simulink model "CCModel_73"  (R2024a)
settings: Solver=ode3  StartTime=0.0  StopTime=100  FixedStep=0.001  RelTol=1e-3  EnableMultiTasking=on
undefined symbols (not defined in the file or in its folder): DiscIntNeverNeededParam, Hecate_desVel1, Hecate_desVel2, Hecate_desVel3, Hecate_horShift, Hecate_period, Hecate_slope, Hecate_Transition1, Hecate_Transition2, Hecate_verShift, i, PME_qb, qb_map, RPM_qb, V
libraries: simulink x46
(part 3 of 11)

== system CCModel_73/Powertrain/EMR ==
  note: If Torque is positive: Motor does its best
      | If torque is negative: Case 01: SOC > 99: No Regen (Tmot = 0)
      | Case 02: SOC < 99: Regen
      | If Vehicle is stopped: No Regen Brakes
  0 : Constant
  "1 " : Constant  Value=0
  EMS Active : Constant  Value=EMRActive
  GEN Ratio : Constant
  Memory1 : Memory  InheritSampleTime=on
  Negative Motor Torque Table : Lookup_n-D  NumberOfTableDimensions=1  BreakpointsForDimension1=|  Table=|  InternalRulePriority=Speed  RndMeth=Simplest
      BreakpointsForDimension1=|
      | [1
      | 300
      | 700
      | 1000
      | 1300
      | 1600
      | 1900
      | 2200
      | 2500
      | 2800
      | 3100
      | 3400
      | 3700
      | 4000
      | 4300
      | 4600
      | 4900
      | 5200
      | 5500
      | 5800
      | 6100
      | 6400
      | 6700
      | 7000
      | 7400
      | 7800
      | 8200
      | 8600
      | 8810]
      Table=|
      | [-360
      | -360
      | -360
      | -360
      | -360
      | -357.728404316261
      | -357.682405078656
      | -356.960983702214
      | -356.300227986961
      | -355.518140949330
      | -355.472141711725
      | -351.285699987009
      | -343.284814075766
      | -334.455149023278
      | -326.397812480700
      | -307.963362459085
      | -289.161940741908
      | -276.934802218937
      | -265.691686602383
      | -254.400604378871
      | -242.676261199004
      | -229.462130210989
      | -218.075437684875
      | -207.776256300937
      | -192.222891861329
      | -178.005775209291
      | -168.578005975641
      | -157.192637101830
      | -152.195121951219]
  Positive Motor Torque Table : Lookup_n-D  NumberOfTableDimensions=1  BreakpointsForDimension1=|  Table=|  InternalRulePriority=Speed  RndMeth=Simplest
      BreakpointsForDimension1=|
      | [1
      | 300
      | 700
      | 1000
      | 1300
      | 1600
      | 1900
      | 2200
      | 2500
      | 2800
      | 3100
      | 3400
      | 3700
      | 4000
      | 4300
      | 4600
      | 4900
      | 5200
      | 5500
      | 5800
      | 6100
      | 6400
      | 6700
      | 7000
      | 7400
      | 7800
      | 8200
      | 8600
      | 8810]
      Table=|
      | [360
      | 360
      | 360
      | 360
      | 360
      | 357.728404316261
      | 357.682405078656
      | 356.960983702214
      | 356.300227986961
      | 355.518140949330
      | 355.472141711725
      | 351.285699987009
      | 343.284814075766
      | 334.455149023278
      | 326.397812480700
      | 307.963362459085
      | 289.161940741908
      | 276.934802218937
      | 265.691686602383
      | 254.400604378871
      | 242.676261199004
      | 229.462130210989
      | 218.075437684875
      | 207.776256300937
      | 192.222891861329
      | 178.005775209291
      | 168.578005975641
      | 157.192637101830
      | 152.195121951219]
  Product : Product
  Saturation Dynamic1 : simulink/Discontinuities/Saturation Dynamic  OutMin=[-360]  OutMax=[360]  OutDataTypeStr=Inherit: Same as second input  OutDataType=fixdt(1, 16)  OutScaling=2^-10  DoSatur=off
  Switch : Switch  Criteria=u2 > Threshold  SaturateOnIntegerOverflow=off  InputSameDT=off
  Switch3 : Switch  SaturateOnIntegerOverflow=off  InputSameDT=off
  efficiency : Subsystem
  prod : Product
  prod1 : Product
  prod2 : Product
  rad_sec_to_rpm : Gain  Gain=60/2/pi
  tag scope: EMRRatio=global, EMRTorque=global, EMR_ElectricPower_W=global, InternalEMRActivity=global
  wires:
  [EMRTorqueCmd] -> Saturation Dynamic1/2
  Switch3/1 -> prod/1
  Positive Motor Torque Table/1 -> Saturation Dynamic1/1
  Product/1 -> [EMRTorque]
  "1 "/1 -> Switch/1
  [EMROutputOmega] -> rad_sec_to_rpm/1
  0/1 -> Switch/3
  prod/1 -> efficiency/2("Torque [Nm] "), Product/1
  EMS Active/1 -> prod1/2, prod/2, Switch/2
  GEN Ratio/1 -> [EMRRatio], Product/2
  Saturation Dynamic1/1 -> prod2/1, Switch3/2, Switch3/1
  Memory1/1 -> Negative Motor Torque Table/1, Positive Motor Torque Table/1
  Negative Motor Torque Table/1 -> Saturation Dynamic1/3
  rad_sec_to_rpm/1 -> efficiency/1(Motor speed [rpm]), Memory1/1
  prod1/1 -> [EMR_ElectricPower_W]
  efficiency/1(Electrical power [W]) -> prod1/1
  Switch/1 -> [InternalEMRActivity]
  [RegenFactor] -> prod2/2
  prod2/1 -> Switch3/3

== system CCModel_73/Powertrain/EMS ==
  note: If Torque is positive: Motor does its best
      | If torque is negative: Case 01: SOC > 99: No Regen (Tmot = 0)
      | Case 02: SOC < 99: Regen
      | If Vehicle is stopped: No Regen Brakes
  0 : Constant
  "1 " : Constant  Value=0
  Constant1 : Constant  Value=0
  EMS Active : Constant  Value=EMSActive
  GEN Ratio : Constant
  Memory1 : Memory  InheritSampleTime=on
  Negative Motor Torque Table : Lookup_n-D  NumberOfTableDimensions=1  BreakpointsForDimension1=|  Table=|  InternalRulePriority=Speed  RndMeth=Simplest
      BreakpointsForDimension1=|
      | [1
      | 300
      | 700
      | 1000
      | 1300
      | 1600
      | 1900
      | 2200
      | 2500
      | 2800
      | 3100
      | 3400
      | 3700
      | 4000
      | 4300
      | 4600
      | 4900
      | 5200
      | 5500
      | 5800
      | 6100
      | 6400
      | 6700
      | 7000
      | 7400
      | 7800
      | 8200
      | 8600
      | 8810]
      Table=|
      | [-360
      | -360
      | -360
      | -360
      | -360
      | -357.728404316261
      | -357.682405078656
      | -356.960983702214
      | -356.300227986961
      | -355.518140949330
      | -355.472141711725
      | -351.285699987009
      | -343.284814075766
      | -334.455149023278
      | -326.397812480700
      | -307.963362459085
      | -289.161940741908
      | -276.934802218937
      | -265.691686602383
      | -254.400604378871
      | -242.676261199004
      | -229.462130210989
      | -218.075437684875
      | -207.776256300937
      | -192.222891861329
      | -178.005775209291
      | -168.578005975641
      | -157.192637101830
      | -152.195121951219]
  Positive Motor Torque Table : Lookup_n-D  NumberOfTableDimensions=1  BreakpointsForDimension1=|  Table=|  InternalRulePriority=Speed  RndMeth=Simplest
      BreakpointsForDimension1=|
      | [1
      | 300
      | 700
      | 1000
      | 1300
      | 1600
      | 1900
      | 2200
      | 2500
      | 2800
      | 3100
      | 3400
      | 3700
      | 4000
      | 4300
      | 4600
      | 4900
      | 5200
      | 5500
      | 5800
      | 6100
      | 6400
      | 6700
      | 7000
      | 7400
      | 7800
      | 8200
      | 8600
      | 8810]
      Table=|
      | [360
      | 360
      | 360
      | 360
      | 360
      | 357.728404316261
      | 357.682405078656
      | 356.960983702214
      | 356.300227986961
      | 355.518140949330
      | 355.472141711725
      | 351.285699987009
      | 343.284814075766
      | 334.455149023278
      | 326.397812480700
      | 307.963362459085
      | 289.161940741908
      | 276.934802218937
      | 265.691686602383
      | 254.400604378871
      | 242.676261199004
      | 229.462130210989
      | 218.075437684875
      | 207.776256300937
      | 192.222891861329
      | 178.005775209291
      | 168.578005975641
      | 157.192637101830
      | 152.195121951219]
  Product : Product
  Saturation Dynamic1 : simulink/Discontinuities/Saturation Dynamic  OutMin=[-360]  OutMax=[360]  OutDataTypeStr=Inherit: Same as second input  OutDataType=fixdt(1, 16)  OutScaling=2^-10  DoSatur=off
  Switch : Switch  Criteria=u2 > Threshold  SaturateOnIntegerOverflow=off  InputSameDT=off
  Switch3 : Switch  SaturateOnIntegerOverflow=off  InputSameDT=off
  compare SOC to SOC _max : Switch  Criteria=u2 > Threshold  Threshold=99  SaturateOnIntegerOverflow=off  InputSameDT=off
  efficiency : Subsystem
  prod : Product
  prod1 : Product
  rad_sec_to_rpm : Gain  Gain=60/2/pi
  tag scope: EMSRatio=global, EMSTorque=global, EMS_ElectricPower_W=global, InternalEMSActivity=global
  wires:
  Switch/1 -> [InternalEMSActivity]
  "1 "/1 -> Switch/1
  0/1 -> Switch/3
  prod/1 -> efficiency/2("Torque [Nm] "), Product/1
  rad_sec_to_rpm/1 -> efficiency/1(Motor speed [rpm]), Memory1/1
  [EMSOutputOmega] -> rad_sec_to_rpm/1
  prod1/1 -> [EMS_ElectricPower_W]
  Negative Motor Torque Table/1 -> Saturation Dynamic1/3
  Product/1 -> [EMSTorque]
  GEN Ratio/1 -> [EMSRatio], Product/2
  Memory1/1 -> Negative Motor Torque Table/1, Positive Motor Torque Table/1
  Switch3/1 -> prod/1
  efficiency/1(Electrical power [W]) -> prod1/1
  Saturation Dynamic1/1 -> Switch3/2, Switch3/1, compare SOC to SOC _max/3
  [SOC] -> compare SOC to SOC _max/2
  compare SOC to SOC _max/1 -> Switch3/3
  Constant1/1 -> compare SOC to SOC _max/1
  Positive Motor Torque Table/1 -> Saturation Dynamic1/1
  EMS Active/1 -> prod1/2, prod/2, Switch/2
  [EMSTorqueCmd] -> Saturation Dynamic1/2

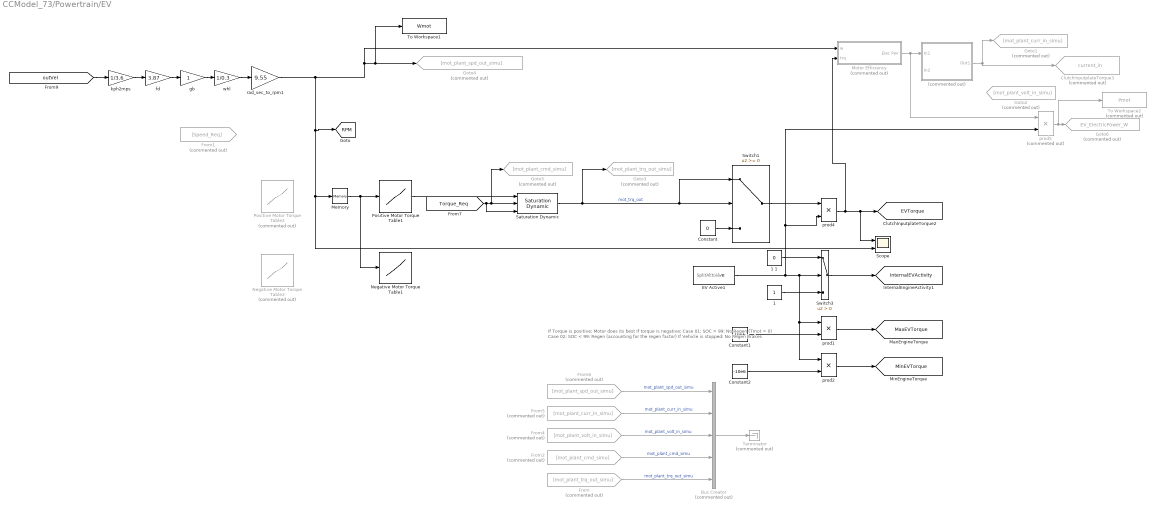
== system CCModel_73/Powertrain/EV ==
  note: If Torque is positive: Motor does its best
      | If torque is negative: Case 01: SOC > 99: No Regen (Tmot = 0)
      | Case 02: SOC < 99: Regen (accounting for the regen factor)
      | If Vehicle is stopped: No Regen Brakes
  note: SplitActive
  " " : Subsystem  Commented=on
      mask Display: fprintf('Divider')
  1 : Constant
  1 1 : Constant  Value=0
  Bus Creator : BusCreator  Commented=on  Inputs='mot_plant_spd_out_simu','mot_plant_curr_in_simu','mot_plant_volt_in_simu','mot_plant_cmd_simu','mot_plant_trq_out_simu'
  ClutchInputplateTorque3 : Goto  Commented=on  GotoTag=current_in  TagVisibility=global
  Constant : Constant  Value=0
  Constant1 : Constant  Value=10e6
  Constant2 : Constant  Value=-10e6
  EV Active1 : Constant  Value=EVActive
  From : From  Commented=on  GotoTag=mot_plant_trq_out_simu
  From1 : From  Commented=on  GotoTag=Speed_Req  TagVisibility=global
  From2 : From  Commented=on  GotoTag=mot_plant_cmd_simu
  From4 : From  Commented=on  GotoTag=mot_plant_volt_in_simu
  From5 : From  Commented=on  GotoTag=mot_plant_curr_in_simu
  From6 : From  Commented=on  GotoTag=mot_plant_spd_out_simu
  Goto1 : Goto  Commented=on  GotoTag=mot_plant_curr_in_simu
  Goto2 : Goto  Commented=on  GotoTag=mot_plant_volt_in_simu
  Goto3 : Goto  Commented=on  GotoTag=mot_plant_trq_out_simu
  Goto4 : Goto  Commented=on  GotoTag=mot_plant_spd_out_simu
  Goto5 : Goto  Commented=on  GotoTag=mot_plant_cmd_simu
  Goto6 : Goto  Commented=on  GotoTag=EV_ElectricPower_W  TagVisibility=global
  Memory : Memory
  Motor Efficiency : Subsystem  Commented=on
  Negative Motor Torque Table1 : Lookup_n-D  NumberOfTableDimensions=1  BreakpointsForDimension1="[5.65\t554.29\t1108.59\t1662.89\t2024.88\t2211.53\t2369.9\t2522.62\t2680.99\t2873.3\t3088.23\t3252.26\t3433.25\t3625.56\t3812.21\t4095.02\t4389.14\t4536.19\t4626.69\t4700.22\t4756.78\t4819\t4869.9\t4920.81\t4977.37\t4999.99]"  Table="[-444\t-444\t-444\t-444\t-428\t-416.41\t-396.47\t-372.36\t-344.93\t-310.84\t-285.92\t-268.48\t-248.55\t-233.62\t-218.68\t-200.45\t-193.05\t-186.44\t-173.14\t-154.84\t-129.037\t-101.56\t-73.26\t-46.62\t-17.48\t0]"  InternalRulePriority=Speed  RndMeth=Simplest
  Negative Motor Torque Table2 : Lookup_n-D  Commented=on  NumberOfTableDimensions=1  BreakpointsForDimension1=[0 5000]  Table=[-500 -500]  InternalRulePriority=Speed  RndMeth=Simplest
  Positive Motor Torque Table1 : Lookup_n-D  NumberOfTableDimensions=1  BreakpointsForDimension1=[1;10;575;750;925;1100;1275;1450;1625;1800;1975;2150;2325;2500;2675;2850;3025;3200;3375;3550;3725;3900;4075;4250;4425;4600;4775;4950;5125;5300;5475;5650;5825;6000]  Table=[412.5;412.5;412.5;412.5;412.5;412.5;412.5;412.5;412.5;412.5;412.5;412.5;412.5;412.5;412.5;412.5;412.5;412.5;412.5;412.5;400;380;355.5626875;346.30825;338.1746875;331.162;325.2701875;320.49925;316.8491875;314.32;308;275;50;0.195]  InternalRulePriority=Speed  RndMeth=Simplest
  Positive Motor Torque Table2 : Lookup_n-D  Commented=on  NumberOfTableDimensions=1  BreakpointsForDimension1=[0 500 1000 1500 2000 2500 3000 3500 4000 4500 5000]  Table=[436 426 416 408 405 330 258 207 172 140 0]  InternalRulePriority=Speed  RndMeth=Simplest
  Saturation Dynamic : simulink/Discontinuities/Saturation Dynamic  OutMin=[-444]  OutMax=[444]  OutDataTypeStr=Inherit: Same as second input  OutDataType=fixdt(1, 16)  OutScaling=2^-10  DoSatur=off
  Scope : Scope  NumInputPorts=2
  Switch1 : Switch  SaturateOnIntegerOverflow=off  InputSameDT=off
  Switch3 : Switch  Criteria=u2 > Threshold  SaturateOnIntegerOverflow=off  InputSameDT=off
  Terminator : Terminator  Commented=on
  To Workspace1 : ToWorkspace  VariableName=Wmot  SampleTime=-1
      settings: Save2DSignal=2-D array (concatenate along first dimension)
  To Workspace2 : ToWorkspace  Commented=on  VariableName=Pmot  SampleTime=-1
      settings: Save2DSignal=2-D array (concatenate along first dimension)
  fd : Gain  Gain=3.87
  gb : Gain
  kph2mps : Gain  Gain=1/3.6
  prod1 : Product
  prod2 : Product
  prod4 : Product
  prod5 : Product  Commented=on
  rad_sec_to_rpm1 : Gain  Gain=9.55
  whl : Gain  Gain=1/0.3
  tag scope: EVTorque=global, InternalEVActivity=global, MaxEVTorque=global, MinEVTorque=global, RPM=global
  wires:
  rad_sec_to_rpm1/1 -> [RPM], Scope/2, Memory/1, Motor Efficiency/1(w), To Workspace1/1, Goto4/1
  Saturation Dynamic/1 -> Switch1/2, Switch1/1, Goto3/1  "mot_trq_out"
  From5/1 -> Bus Creator/2  "mot_plant_curr_in_simu"
  [Torque_Req] -> Saturation Dynamic/3, Goto5/1, Saturation Dynamic/2
  From/1 -> Bus Creator/5  "mot_plant_trq_out_simu"
  Bus Creator/1 -> Terminator/1
  From6/1 -> Bus Creator/1  "mot_plant_spd_out_simu"
  Memory/1 -> Negative Motor Torque Table1/1, Positive Motor Torque Table1/1
  Positive Motor Torque Table1/1 -> Saturation Dynamic/1
  From2/1 -> Bus Creator/4  "mot_plant_cmd_simu"
  From4/1 -> Bus Creator/3  "mot_plant_volt_in_simu"
  [outVel] -> kph2mps/1
  1 1/1 -> Switch3/1
  Switch3/1 -> [InternalEVActivity]
  1/1 -> Switch3/3
  Switch1/1 -> prod4/1
  prod5/1 -> To Workspace2/1, Goto6/1
  Motor Efficiency/1(Elec Pwr) -> prod5/1, " "/1(In1)
  " "/1(Out1) -> ClutchInputplateTorque3/1, Goto1/1
  Constant2/1 -> prod2/2
  EV Active1/1 -> prod5/2, prod4/2, prod1/1, prod2/1, Switch3/2
  Constant1/1 -> prod1/2
  fd/1 -> gb/1
  gb/1 -> whl/1
  kph2mps/1 -> fd/1
  whl/1 -> rad_sec_to_rpm1/1
  prod4/1 -> Motor Efficiency/2(trq), Scope/1, [EVTorque]
  prod1/1 -> [MaxEVTorque]
  prod2/1 -> [MinEVTorque]
  Constant/1 -> Switch1/3

== system CCModel_73/Powertrain/Engine ==
  1 2 : Constant  Value=0
  2 : Constant
  Constant1 : Constant  Value=10e6
  Constant2 : Constant  Value=-10e6
  Eengine Active : Constant  Value=EngineActive
  EngineOmega : Goto  Commented=on  GotoTag=EngineOmega  TagVisibility=global
  Fuel Consumption : Subsystem  Commented=on
      mask Display: image(imread('engine_icon.jpg'))
  ICE_WOT : Lookup_n-D  NumberOfTableDimensions=1  BreakpointsForDimension1=[0 1500 2000 2500 3000 3500 4000 4500 5000 5500 6000 6500 7000 7200]  Table=[0 460 475 490 500 510 530 540 530 510 480 455 420 400]  InternalRulePriority=Speed  RndMeth=Simplest
  IdleSpeed(rpm) : Constant  Value=IdleSpeed
  Idle_Speed : Saturate  UpperLimit=inf  LowerLimit=800
  Idle_if_N : Switch  Criteria=u2 > Threshold  SaturateOnIntegerOverflow=off  InputSameDT=off
  Memory18 : Memory  InheritSampleTime=on
  Memory2 : Memory  InheritSampleTime=on
  Min : MinMax  Inputs=2
  Product6 : Product
  Saturation : Saturate  UpperLimit=inf  LowerLimit=0
  Switch1 : Switch  Criteria=u2 > Threshold  SaturateOnIntegerOverflow=off  InputSameDT=off
  prod{1..4} (4 alike) : Product
  rad_sec_to_rpm2 : Gain  Gain=60/2/pi
  rpm_to_radsec : Gain  Gain=1/(60/2/pi)
  tag scope: ClutchInputplateTorque=global, InternalEngineActivity=global, MaxEngineTorque=global, MinEngineTorque=global
  wires:
  Constant1/1 -> prod1/2
  Constant2/1 -> prod2/2
  [EngineTorqueCmd] -> Min/1
  prod3/1 -> [ClutchInputplateTorque]
  Eengine Active/1 -> prod4/2, prod3/2, prod2/1, prod1/1, Switch1/2
  ICE_WOT/1 -> Min/2
  1 2/1 -> Switch1/1
  2/1 -> Switch1/3
  rad_sec_to_rpm2/1 -> Memory2/1
  Switch1/1 -> [InternalEngineActivity]
  Saturation/1 -> prod3/1
  Min/1 -> Saturation/1
  Idle_Speed/1 -> ICE_WOT/1
  Memory2/1 -> Idle_Speed/1
  Memory18/1 -> prod4/1, rad_sec_to_rpm2/1
  prod1/1 -> [MaxEngineTorque]
  prod2/1 -> [MinEngineTorque]
  [DiffCenterInputOmega] -> Product6/2
  [GearRatio] -> Idle_if_N/2, Product6/1
  Product6/1 -> Idle_if_N/1
  prod4/1 -> EngineOmega/1
  Idle_if_N/1 -> Memory18/1
  IdleSpeed(rpm)/1 -> rpm_to_radsec/1
  rpm_to_radsec/1 -> Idle_if_N/3

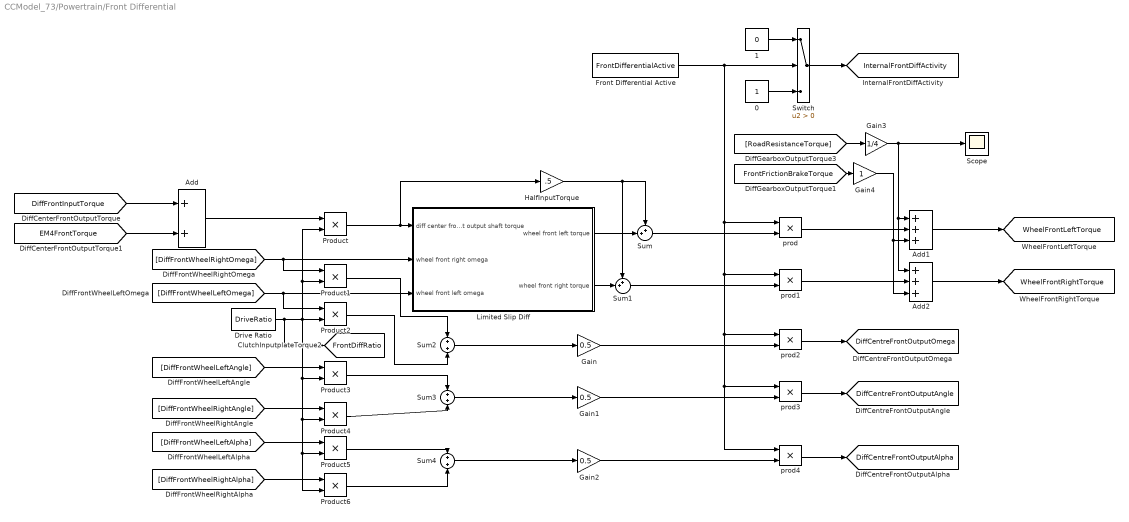
== system CCModel_73/Powertrain/Front Differential ==
  0 : Constant
  "1 " : Constant  Value=0
  Add : Sum
  Add1 : Sum  Inputs=+++
  Add2 : Sum  Inputs=+++
  Drive Ratio : Constant  Value=DriveRatio
  Front Differential Active : Constant  Value=FrontDifferentialActive
  Gain : Gain  Gain=0.5
  Gain1 : Gain  Gain=0.5
  Gain2 : Gain  Gain=0.5
  Gain3 : Gain  Gain=1/4
  Gain4 : Gain
  HalfInputTorque : Gain  Gain=.5
  Limited Slip Diff : Subsystem  mask{C0=0, C1=.05, C2=.8, C3=.5}
  Product{,1..6} (7 alike) : Product
  Scope : Scope
  Sum : Sum  Inputs=++|
  Sum1 : Sum  Inputs=++|
  Sum2 : Sum
  Sum3 : Sum
  Sum4 : Sum
  Switch : Switch  Criteria=u2 > Threshold  SaturateOnIntegerOverflow=off  InputSameDT=off
  prod{,1..4} (5 alike) : Product
  tag scope: DiffCentreFrontOutputAlpha=global, DiffCentreFrontOutputAngle=global, DiffCentreFrontOutputOmega=global, FrontDiffRatio=global, InternalFrontDiffActivity=global, WheelFrontLeftTorque=global, WheelFrontRightTorque=global
  wires:
  [DiffFrontWheelRightAngle] -> Product4/1
  [DiffFrontWheelLeftAlpha] -> Product5/1
  [DiffFrontWheelLeftAngle] -> Product3/1
  Sum2/1 -> Gain/1
  [DiffFrontWheelRightOmega] -> Limited Slip Diff/2(wheel front right omega), Product1/1
  [DiffFrontWheelLeftOmega] -> Limited Slip Diff/3(wheel front left omega), Product2/1
  [DiffFrontInputTorque] -> Add/1
  HalfInputTorque/1 -> Sum/1, Sum1/1
  Sum3/1 -> Gain1/1
  [DiffFrontWheelRightAlpha] -> Product6/1
  Sum4/1 -> Gain2/1
  Limited Slip Diff/1(wheel front left torque) -> Sum/2
  Limited Slip Diff/2(wheel front right torque) -> Sum1/2
  Product/1 -> HalfInputTorque/1, Limited Slip Diff/1(diff center front output shaft torque)
  Product1/1 -> Sum2/1
  Product2/1 -> Sum2/2
  Product3/1 -> Sum3/1
  Product4/1 -> Sum3/2
  Product5/1 -> Sum4/1
  Product6/1 -> Sum4/2
  Drive Ratio/1 -> [FrontDiffRatio], Product6/2, Product5/2, Product4/2, Product3/2, Product/2, Product1/2, Product2/2
  prod/1 -> Add1/2
  prod1/1 -> Add2/2
  prod2/1 -> [DiffCentreFrontOutputOmega]
  prod3/1 -> [DiffCentreFrontOutputAngle]
  prod4/1 -> [DiffCentreFrontOutputAlpha]
  Sum/1 -> prod/2
  Sum1/1 -> prod1/2
  Gain/1 -> prod2/2
  Gain1/1 -> prod3/2
  Gain2/1 -> prod4/2
  Front Differential Active/1 -> prod4/1, prod3/1, prod2/1, prod1/1, prod/1, Switch/2
  Switch/1 -> [InternalFrontDiffActivity]
  "1 "/1 -> Switch/1
  0/1 -> Switch/3
  [EM4FrontTorque] -> Add/2
  Add/1 -> Product/1
  [RoadResistanceTorque] -> Gain3/1
  Gain3/1 -> Scope/1, Add2/1, Add1/1
  Gain4/1 -> Add2/3, Add1/3
  [FrontFrictionBrakeTorque] -> Gain4/1
  Add1/1 -> [WheelFrontLeftTorque]
  Add2/1 -> [WheelFrontRightTorque]

== system CCModel_73/Powertrain/GEN ==
  note: If Torque is positive: Motor does its best
      | If torque is negative: Case 01: SOC > 99: No Regen (Tmot = 0)
      | Case 02: SOC < 99: Regen
      | If Vehicle is stopped: No Regen Brakes
  0 : Constant
  "1 " : Constant  Value=0
  Constant1 : Constant  Value=0
  GEN Active : Constant  Value=GENActive
  GEN Ratio : Constant
  Memory1 : Memory  InheritSampleTime=on
  Negative Motor Torque Table : Lookup_n-D  NumberOfTableDimensions=1  BreakpointsForDimension1=|  Table=|  InternalRulePriority=Speed  RndMeth=Simplest
      BreakpointsForDimension1=|
      | [1
      | 300
      | 700
      | 1000
      | 1300
      | 1600
      | 1900
      | 2200
      | 2500
      | 2800
      | 3100
      | 3400
      | 3700
      | 4000
      | 4300
      | 4600
      | 4900
      | 5200
      | 5500
      | 5800
      | 6100
      | 6400
      | 6700
      | 7000
      | 7400
      | 7800
      | 8200
      | 8600
      | 8810]
      Table=|
      | [-360
      | -360
      | -360
      | -360
      | -360
      | -357.728404316261
      | -357.682405078656
      | -356.960983702214
      | -356.300227986961
      | -355.518140949330
      | -355.472141711725
      | -351.285699987009
      | -343.284814075766
      | -334.455149023278
      | -326.397812480700
      | -307.963362459085
      | -289.161940741908
      | -276.934802218937
      | -265.691686602383
      | -254.400604378871
      | -242.676261199004
      | -229.462130210989
      | -218.075437684875
      | -207.776256300937
      | -192.222891861329
      | -178.005775209291
      | -168.578005975641
      | -157.192637101830
      | -152.195121951219]
  Positive Motor Torque Table : Lookup_n-D  NumberOfTableDimensions=1  BreakpointsForDimension1=|  Table=|  InternalRulePriority=Speed  RndMeth=Simplest
      BreakpointsForDimension1=|
      | [1
      | 300
      | 700
      | 1000
      | 1300
      | 1600
      | 1900
      | 2200
      | 2500
      | 2800
      | 3100
      | 3400
      | 3700
      | 4000
      | 4300
      | 4600
      | 4900
      | 5200
      | 5500
      | 5800
      | 6100
      | 6400
      | 6700
      | 7000
      | 7400
      | 7800
      | 8200
      | 8600
      | 8810]
      Table=|
      | [360
      | 360
      | 360
      | 360
      | 360
      | 357.728404316261
      | 357.682405078656
      | 356.960983702214
      | 356.300227986961
      | 355.518140949330
      | 355.472141711725
      | 351.285699987009
      | 343.284814075766
      | 334.455149023278
      | 326.397812480700
      | 307.963362459085
      | 289.161940741908
      | 276.934802218937
      | 265.691686602383
      | 254.400604378871
      | 242.676261199004
      | 229.462130210989
      | 218.075437684875
      | 207.776256300937
      | 192.222891861329
      | 178.005775209291
      | 168.578005975641
      | 157.192637101830
      | 152.195121951219]
  Product : Product
  Saturation Dynamic1 : simulink/Discontinuities/Saturation Dynamic  OutMin=[-360]  OutMax=[360]  OutDataTypeStr=Inherit: Same as second input  OutDataType=fixdt(1, 16)  OutScaling=2^-10  DoSatur=off
  Switch : Switch  Criteria=u2 > Threshold  SaturateOnIntegerOverflow=off  InputSameDT=off
  Switch3 : Switch  SaturateOnIntegerOverflow=off  InputSameDT=off
  compare SOC to SOC _max : Switch  Criteria=u2 > Threshold  Threshold=99  SaturateOnIntegerOverflow=off  InputSameDT=off
  efficiency : Subsystem
  prod : Product
  prod1 : Product
  rad_sec_to_rpm : Gain  Gain=60/2/pi
  tag scope: GENRatio=global, GENTorque=global, GEN_ElectricPower_W=global, InternalGENActivity=global
  wires:
  Switch/1 -> [InternalGENActivity]
  "1 "/1 -> Switch/1
  0/1 -> Switch/3
  GEN Active/1 -> prod1/2, prod/2, Switch/2
  Memory1/1 -> Negative Motor Torque Table/1, Positive Motor Torque Table/1
  [GENTorqueCmd] -> Saturation Dynamic1/2
  efficiency/1(Electrical power [W]) -> prod1/1
  Constant1/1 -> compare SOC to SOC _max/1
  Saturation Dynamic1/1 -> Switch3/2, Switch3/1, compare SOC to SOC _max/3
  [GENOmega] -> rad_sec_to_rpm/1
  compare SOC to SOC _max/1 -> Switch3/3
  Positive Motor Torque Table/1 -> Saturation Dynamic1/1
  Switch3/1 -> prod/1
  [SOC] -> compare SOC to SOC _max/2
  Negative Motor Torque Table/1 -> Saturation Dynamic1/3
  rad_sec_to_rpm/1 -> efficiency/1(Motor speed [rpm]), Memory1/1
  prod1/1 -> [GEN_ElectricPower_W]
  prod/1 -> efficiency/2("Torque [Nm] "), Product/1
  GEN Ratio/1 -> [GENRatio], Product/2
  Product/1 -> [GENTorque]

== system CCModel_73/Powertrain/Gearbox ==
  "      " : Product  Inputs=**
  " " : Product  Inputs=**
  "        " : Product  Inputs=**
  "      1" : Product  Inputs=**
  0 : Constant
  "1 " : Constant  Value=0
  AT_Active : Constant  Value=AT
  Add : Sum  Inputs=+++
  Final Drive : Gain
  Gear Ratio1 : Lookup  InputValues=[0 1 2 3 4 5 6 7]  Table=[0 3.788 2.05 1.276 0.941 0.692 0.571 0.45]  SaturateOnIntegerOverflow=off
  Gearbox Active : Constant  Value=GearboxActive
  MT_or_AT : Switch  Criteria=u2 > Threshold  SaturateOnIntegerOverflow=off  InputSameDT=off
  Switch : Switch  Criteria=u2 > Threshold  SaturateOnIntegerOverflow=off  InputSameDT=off
  prod{,1..3} (4 alike) : Product
  tag scope: ClutchOutputplateAlpha=global, ClutchOutputplateAngle=global, ClutchOutputplateOmega=global, DiffCenterInputshaftTorque=global, GearEngaged=global, GearRatio=global, InternalGearboxActivity=global
  wires:
  Gear Ratio1/1 -> [GearRatio], Final Drive/1
  [GearboxInputTorque] -> Add/1
  [DiffCenterInputOmega] -> "      "/1
  [DiffCenterInputAngle] -> "      1"/1
  [DiffCenterInputAlpha] -> " "/1
  Final Drive/1 -> "      1"/2, " "/2, "      "/2, "        "/2
  Gearbox Active/1 -> Switch/2, prod3/1, prod2/1, prod1/1, prod/1
  prod/1 -> [ClutchOutputplateAlpha]
  " "/1 -> prod/2
  "      1"/1 -> prod1/2
  "      "/1 -> prod2/2
  "        "/1 -> prod3/2
  prod1/1 -> [ClutchOutputplateAngle]
  prod2/1 -> [ClutchOutputplateOmega]
  prod3/1 -> [DiffCenterInputshaftTorque]
  Switch/1 -> [InternalGearboxActivity]
  "1 "/1 -> Switch/1
  0/1 -> Switch/3
  Add/1 -> "        "/1
  [EM2Torque] -> Add/2
  [MOTTorque] -> Add/3
  AT_Active/1 -> MT_or_AT/2
  [GearDemandAT] -> MT_or_AT/1
  MT_or_AT/1 -> [GearEngaged]
  [GearEngaged] -> Gear Ratio1/1
  [GearDemandMT] -> MT_or_AT/3

== system CCModel_73/Powertrain/MOT ==
  note: If Torque is positive: Motor does its best
      | If torque is negative: Case 01: SOC > 99: No Regen (Tmot = 0)
      | Case 02: SOC < 99: Regen
      | If Vehicle is stopped: No Regen Brakes
  0 : Constant
  "1 " : Constant  Value=0
  Add : Sum
  Belt_Ratio : Gain
  Constant : Constant  Value=0
  MOT Active : Constant  Value=MOTActive
  Memory2 : Memory  InheritSampleTime=on
  Negative Motor Torque Table1 : Lookup_n-D  NumberOfTableDimensions=1  BreakpointsForDimension1=|  Table=|  InternalRulePriority=Speed  RndMeth=Simplest
      BreakpointsForDimension1=|
      | [1
      | 300
      | 700
      | 1000
      | 1300
      | 1600
      | 1900
      | 2200
      | 2500
      | 2800
      | 3100
      | 3400
      | 3700
      | 4000
      | 4300
      | 4600
      | 4900
      | 5200
      | 5500
      | 5800
      | 6100
      | 6400
      | 6700
      | 7000
      | 7400
      | 7800
      | 8200
      | 8600
      | 8810]
      Table=|
      | [-360
      | -360
      | -360
      | -360
      | -360
      | -357.728404316261
      | -357.682405078656
      | -356.960983702214
      | -356.300227986961
      | -355.518140949330
      | -355.472141711725
      | -351.285699987009
      | -343.284814075766
      | -334.455149023278
      | -326.397812480700
      | -307.963362459085
      | -289.161940741908
      | -276.934802218937
      | -265.691686602383
      | -254.400604378871
      | -242.676261199004
      | -229.462130210989
      | -218.075437684875
      | -207.776256300937
      | -192.222891861329
      | -178.005775209291
      | -168.578005975641
      | -157.192637101830
      | -152.195121951219]
  Positive Motor Torque Table1 : Lookup_n-D  NumberOfTableDimensions=1  BreakpointsForDimension1=|  Table=|  InternalRulePriority=Speed  RndMeth=Simplest
      BreakpointsForDimension1=|
      | [0
      | 300
      | 700
      | 1000
      | 1300
      | 1600
      | 1900
      | 2200
      | 2500
      | 2800
      | 3100
      | 3400
      | 3700
      | 4000
      | 4300
      | 4600
      | 4900
      | 5200
      | 5500
      | 5800
      | 6100
      | 6400
      | 6700
      | 7000
      | 7400
      | 7800
      | 8200
      | 8600
      | 8810]
      Table=|
      | [360
      | 360
      | 360
      | 360
      | 360
      | 357.728404316261
      | 357.682405078656
      | 356.960983702214
      | 356.300227986961
      | 355.518140949330
      | 355.472141711725
      | 351.285699987009
      | 343.284814075766
      | 334.455149023278
      | 326.397812480700
      | 307.963362459085
      | 289.161940741908
      | 276.934802218937
      | 265.691686602383
      | 254.400604378871
      | 242.676261199004
      | 229.462130210989
      | 218.075437684875
      | 207.776256300937
      | 192.222891861329
      | 178.005775209291
      | 168.578005975641
      | 157.192637101830
      | 152.195121951219]
  Product1 : Product
  Product2 : Product
  Saturation Dynamic2 : simulink/Discontinuities/Saturation Dynamic  OutMin=[-360]  OutMax=[360]  OutDataTypeStr=Inherit: Same as second input  OutDataType=fixdt(1, 16)  OutScaling=2^-10  DoSatur=off
  Switch : Switch  Criteria=u2 > Threshold  SaturateOnIntegerOverflow=off  InputSameDT=off
  Switch1 : Switch  Criteria=u2 > Threshold  Threshold=8810  SaturateOnIntegerOverflow=off  InputSameDT=off
  Switch3 : Switch  SaturateOnIntegerOverflow=off  InputSameDT=off
  decimal : Gain  Gain=0.01
  decimal1 : Gain  Gain=-0.01
  efficiency : Subsystem
  prod : Product
  prod1 : Product
  prod2 : Product
  rad_sec_to_rpm1 : Gain  Gain=60/2/pi
  tag scope: InternalMOTActivity=global, MOTTorque=global, MOT_ElectricPower_W=global
  wires:
  Switch/1 -> [InternalMOTActivity]
  "1 "/1 -> Switch/1
  0/1 -> Switch/3
  MOT Active/1 -> prod1/2, prod/2, Switch/2
  efficiency/1(Electrical power [W]) -> prod1/1
  Saturation Dynamic2/1 -> prod2/1, Switch3/2, Switch3/1
  Switch3/1 -> prod/1
  prod1/1 -> [MOT_ElectricPower_W]
  prod/1 -> efficiency/2("Torque [Nm] "), Belt_Ratio/1
  Belt_Ratio/1 -> [MOTTorque]
  [RegenFactor] -> prod2/2
  prod2/1 -> Switch3/3
  decimal1/1 -> Product2/1
  Product2/1 -> Add/2
  Memory2/1 -> Negative Motor Torque Table1/1, Positive Motor Torque Table1/1
  rad_sec_to_rpm1/1 -> efficiency/1(Motor speed [rpm]), Memory2/1, Switch1/2
  [BrakeCmd] -> decimal1/1
  Product1/1 -> Add/1
  decimal/1 -> Product1/1
  [ThrottleCmd] -> Switch1/3
  Constant/1 -> Switch1/1
  [MOTOmega] -> rad_sec_to_rpm1/1
  Positive Motor Torque Table1/1 -> Saturation Dynamic2/1, Product1/2
  Add/1 -> Saturation Dynamic2/2
  Negative Motor Torque Table1/1 -> Product2/2, Saturation Dynamic2/3
  Switch1/1 -> decimal/1

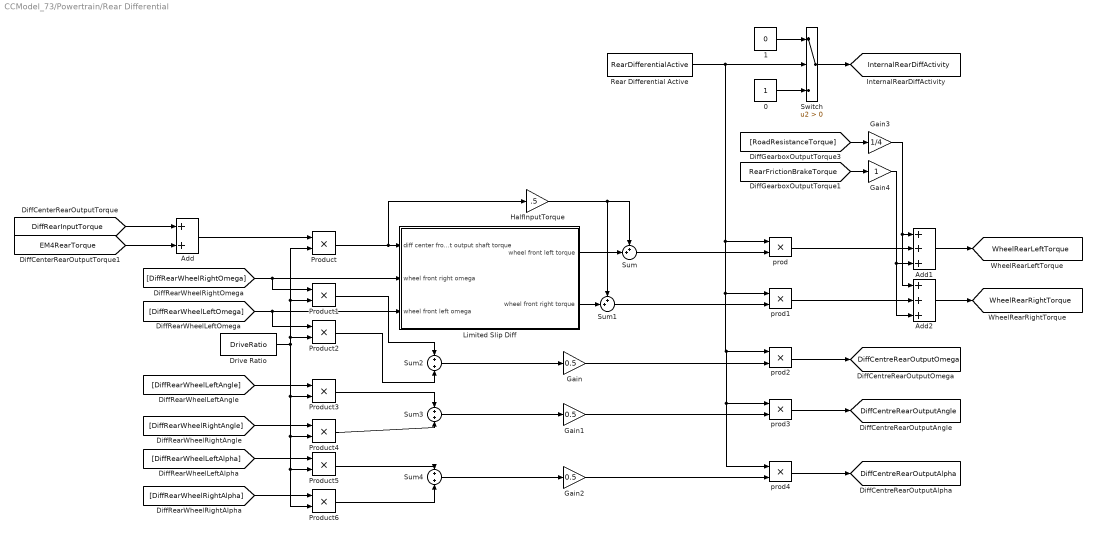
== system CCModel_73/Powertrain/Rear Differential ==
  0 : Constant
  "1 " : Constant  Value=0
  Add : Sum
  Add1 : Sum  Inputs=+++
  Add2 : Sum  Inputs=+++
  Drive Ratio : Constant  Value=DriveRatio
  Gain : Gain  Gain=0.5
  Gain1 : Gain  Gain=0.5
  Gain2 : Gain  Gain=0.5
  Gain3 : Gain  Gain=1/4
  Gain4 : Gain
  HalfInputTorque : Gain  Gain=.5
  Limited Slip Diff : Subsystem  mask{C0=0, C1=.05, C2=.8, C3=.5}
  Product{,1..6} (7 alike) : Product
  Rear Differential Active : Constant  Value=RearDifferentialActive
  Sum : Sum  Inputs=++|
  Sum1 : Sum  Inputs=++|
  Sum2 : Sum
  Sum3 : Sum
  Sum4 : Sum
  Switch : Switch  Criteria=u2 > Threshold  SaturateOnIntegerOverflow=off  InputSameDT=off
  prod{,1..4} (5 alike) : Product
  tag scope: DiffCentreRearOutputAlpha=global, DiffCentreRearOutputAngle=global, DiffCentreRearOutputOmega=global, InternalRearDiffActivity=global, WheelRearLeftTorque=global, WheelRearRightTorque=global
  wires:
  [DiffRearWheelRightAngle] -> Product4/1
  [DiffRearWheelLeftAlpha] -> Product5/1
  [DiffRearWheelLeftAngle] -> Product3/1
  Sum2/1 -> Gain/1
  [DiffRearWheelRightOmega] -> Limited Slip Diff/2(wheel front right omega), Product1/1
  [DiffRearWheelLeftOmega] -> Limited Slip Diff/3(wheel front left omega), Product2/1
  [DiffRearInputTorque] -> Add/1
  HalfInputTorque/1 -> Sum/1, Sum1/1
  Sum3/1 -> Gain1/1
  [DiffRearWheelRightAlpha] -> Product6/1
  Sum4/1 -> Gain2/1
  Limited Slip Diff/1(wheel front left torque) -> Sum/2
  Limited Slip Diff/2(wheel front right torque) -> Sum1/2
  Product/1 -> Limited Slip Diff/1(diff center front output shaft torque), HalfInputTorque/1
  Product1/1 -> Sum2/1
  Product2/1 -> Sum2/2
  Product3/1 -> Sum3/1
  Product4/1 -> Sum3/2
  Product5/1 -> Sum4/1
  Product6/1 -> Sum4/2
  Drive Ratio/1 -> Product6/2, Product5/2, Product4/2, Product3/2, Product/2, Product1/2, Product2/2
  Rear Differential Active/1 -> Switch/2, prod4/1, prod3/1, prod2/1, prod1/1, prod/1
  Add1/1 -> [WheelRearLeftTorque]
  Sum/1 -> prod/2
  Sum1/1 -> prod1/2
  Gain/1 -> prod2/2
  prod2/1 -> [DiffCentreRearOutputOmega]
  Gain1/1 -> prod3/2
  prod3/1 -> [DiffCentreRearOutputAngle]
  prod4/1 -> [DiffCentreRearOutputAlpha]
  Gain2/1 -> prod4/2
  Switch/1 -> [InternalRearDiffActivity]
  "1 "/1 -> Switch/1
  0/1 -> Switch/3
  Add/1 -> Product/1
  [EM4RearTorque] -> Add/2
  [RoadResistanceTorque] -> Gain3/1
  Gain3/1 -> Add2/1, Add1/1
  prod/1 -> Add1/2
  Add2/1 -> [WheelRearRightTorque]
  prod1/1 -> Add2/2
  [RearFrictionBrakeTorque] -> Gain4/1
  Gain4/1 -> Add2/3, Add1/3

== system CCModel_73/Powertrain/Split Device ==
  note: SplitActive
  note: Torque from carrier
  note: em1_spd
  note: clutch
  0 : Constant
  "1 " : Constant  Value=0
  Constant3 : Constant
  Constant4 : Constant
  Constant5 : Constant  Value=0
  Divide : Product  Inputs=*/
  Divide1 : Product  Inputs=*/
  Divide2 : Product  Inputs=*/
  Gain : Gain  Gain=-1
  Power Split Active : Constant  Value=SplitActive
  Product{,1..5} (6 alike) : Product
  Ring2SunRatio : Constant  Value=Ring2Sun
  Ring2SunRatio1 : Constant  Value=Ring2Sun
  Ring2SunRatio2 : Constant  Value=Ring2Sun
  Sum{,1,3..4} (4 alike) : Sum  Inputs=|++
  Sum2 : Sum  Inputs=|+-
  Switch : Switch  Criteria=u2 > Threshold  SaturateOnIntegerOverflow=off  InputSameDT=off
  Switch1 : Switch  Criteria=u2 > Threshold  SaturateOnIntegerOverflow=off  InputSameDT=off
  tag scope: CarrierOmega=global, InternalSplitActivity=global, RingTorque=global, SunTorque=global
  wires:
  Power Split Active/1 -> Product3/2, Product5/2, Product4/2, Switch/2
  Switch/1 -> [InternalSplitActivity]
  "1 "/1 -> Switch/1
  0/1 -> Switch/3
  Divide1/1 -> Product3/1
  [RingOutputOmega] -> Product1/1
  [ClutchCmd] -> Switch1/2
  Constant4/1 -> Sum3/2
  Sum2/1 -> Divide1/1
  Sum/1 -> Product5/1
  Ring2SunRatio1/1 -> Divide2/2
  Constant3/1 -> Sum1/2
  Product2/1 -> Sum2/1
  Product1/1 -> Sum4/2, Sum2/2
  Sum3/1 -> Product2/2, Divide1/2
  Divide/1 -> Product/1
  Sum1/1 -> Divide/2
  Constant5/1 -> Switch1/3
  Product/1 -> Switch1/1, Divide2/1
  [RingTorqueCmd] -> Sum/1
  Switch1/1 -> Sum/2
  Sum4/1 -> Product2/1
  Ring2SunRatio/1 -> Sum1/1, Divide/1
  [EMSOutputOmega] -> Sum4/1
  [EngineTorque] -> Product/2
  Divide2/1 -> Gain/1
  Ring2SunRatio2/1 -> Product1/2, Sum3/1
  Product3/1 -> [CarrierOmega]
  Gain/1 -> Product4/1
  Product4/1 -> [SunTorque]
  Product5/1 -> [RingTorque]

== system CCModel_73/Cruise Control/Version 1.0/PID Controller ==
  error : Inport
  Derivative : Derivative
  Integrator : Integrator
  Kd : Gain  Gain=0.1
  Ki : Gain  Gain=0.03
  Kp : Gain  Gain=3
  Saturation : Saturate  UpperLimit=100  LowerLimit=-100
  Sum : Sum  Inputs=+++
  u : Outport
  wires:
  Integrator/1 -> Ki/1
  error/1 -> Integrator/1, Kp/1, Derivative/1
  Derivative/1 -> Kd/1  "D"
  Sum/1 -> Saturation/1
  Kp/1 -> Sum/2  "P"
  Ki/1 -> Sum/1  "I"
  Kd/1 -> Sum/3
  Saturation/1 -> u/1

== system CCModel_73/Cruise Control/Version 2.0//2.1/PID Controller ==
  error : Inport
  Derivative : Derivative
  Integrator : Integrator
  Kd : Gain  Gain=0.1
  Ki : Gain  Gain=0.03
  Kp : Gain  Gain=9
  Saturation : Saturate  UpperLimit=100  LowerLimit=-100
  Sum : Sum  Inputs=+++
  u : Outport
  wires:
  Integrator/1 -> Ki/1
  error/1 -> Integrator/1, Kp/1, Derivative/1
  Derivative/1 -> Kd/1  "D"
  Sum/1 -> Saturation/1
  Kp/1 -> Sum/2  "P"
  Ki/1 -> Sum/1  "I"
  Kd/1 -> Sum/3
  Saturation/1 -> u/1

== system CCModel_73/Cruise Control/Version 2.0//2.1/Switches ==
  throttle_const : Inport
  u : Inport  Port=2
  brake_const : Inport  Port=3
  (False) : Constant  Value=0
  (True) : Constant
  Brake_Switch : Switch  Criteria=u2 > Threshold  SaturateOnIntegerOverflow=off  InputSameDT=off
  Brake_Switch2 : Switch  Criteria=u2 > Threshold  SaturateOnIntegerOverflow=off  InputSameDT=off
  Constant3 : Constant  Value=0
  Max : MinMax  Function=max  Inputs=2
  Max Brake : Gain  Gain=-1
  Max Throttle : Gain
  Pedal_threshold : Constant  Value=5
  Subtract : Sum  Inputs=+-
  Switch : Switch  Criteria=u2 > Threshold  SaturateOnIntegerOverflow=off  InputSameDT=off
  Throttle_Switch : Switch  Criteria=u2 > Threshold  SaturateOnIntegerOverflow=off  InputSameDT=off
  Throttle_Switch2 : Switch  Criteria=u2 > Threshold  SaturateOnIntegerOverflow=off  InputSameDT=off
  Throttle : Outport
  Brake : Outport  Port=2
  Source : Outport  Port=3
  wires:
  throttle_const/1 -> Max/1, Throttle_Switch2/1
  brake_const/1 -> Max/2, Brake_Switch2/1
  Max/1 -> Subtract/1
  Pedal_threshold/1 -> Subtract/2
  Subtract/1 -> Switch/2
  (True)/1 -> Switch/1
  (False)/1 -> Switch/3
  Switch/1 -> Brake_Switch2/2, Throttle_Switch2/2, Source/1
  u/1 -> Throttle_Switch/2, Max Brake/1, Brake_Switch/2, Max Throttle/1
  Constant3/1 -> Brake_Switch/1, Throttle_Switch/3
  Max Brake/1 -> Brake_Switch/3
  Throttle_Switch/1 -> Throttle_Switch2/3
  Throttle_Switch2/1 -> Throttle/1
  Brake_Switch2/1 -> Brake/1
  Brake_Switch/1 -> Brake_Switch2/3
  Max Throttle/1 -> Throttle_Switch/1

== system CCModel_73/Cruise Control/Version 3.0//3.1//3.2/Detect Change ==
  desired_velocity : Inport
  throttle_const : Inport  Port=2
  brake_const : Inport  Port=3
  u : Inport  Port=4
  (False) : Constant  Value=0
  (True) : Constant
  AND : Logic  IconShape=distinctive  AllPortsSameDT=off  OutDataTypeStr=boolean
  Clock : Clock
  Delay : Delay  DelayLength=1
  Detect Change : simulink/Logic and Bit Operations/Detect Change  vinit=0  OutDataTypeStr=boolean
  Detect Change1 : simulink/Logic and Bit Operations/Detect Change  vinit=0  OutDataTypeStr=boolean
  Max : MinMax  Function=max  Inputs=2
  OR : Logic  Operator=OR  IconShape=distinctive  AllPortsSameDT=off  OutDataTypeStr=boolean
  Pedal_threshold : Constant  Value=5
  Subtract : Sum  Inputs=+-
  Switch : Switch  Criteria=u2 > Threshold  SaturateOnIntegerOverflow=off  InputSameDT=off
  Switch1 : Switch  Criteria=u2 > Threshold  SaturateOnIntegerOverflow=off  InputSameDT=off
  Switch2 : Switch  Criteria=u2 > Threshold  SaturateOnIntegerOverflow=off  InputSameDT=off
  New u : Outport
  wires:
  desired_velocity/1 -> Detect Change/1
  Detect Change/1 -> OR/1
  OR/1 -> Switch/2, Switch2/2
  Switch/1 -> Switch/3
  Switch1/1 -> Detect Change1/1, AND/1
  Detect Change1/1 -> AND/2
  AND/1 -> OR/2
  Clock/1 -> Switch/1
  Max/1 -> Subtract/1
  (True)/1 -> Switch1/1
  brake_const/1 -> Max/2
  Pedal_threshold/1 -> Subtract/2
  Subtract/1 -> Switch1/2
  (False)/1 -> Switch1/3
  throttle_const/1 -> Max/1
  u/1 -> Delay/1, New u/1
  Switch2/1 -> Switch2/3
  Delay/1 -> Switch2/1

== system CCModel_73/Cruise Control/Version 3.0//3.1//3.2/PID Controller ==
  note: Typical PID controller, outputs a value between -100 and 100
  error : Inport
  Derivative : Derivative
  Integrator : Integrator
  Kd : Gain  Gain=0.1
  Ki : Gain  Gain=0.02
  Kp : Gain  Gain=4
  Saturation : Saturate  Commented=through  UpperLimit=200  LowerLimit=-200
  Sum : Sum  Inputs=+++
  u : Outport
  wires:
  Integrator/1 -> Ki/1
  error/1 -> Integrator/1, Kp/1, Derivative/1  "D"
  Kp/1 -> Sum/2  "P"
  Ki/1 -> Sum/1  "I"
  Derivative/1 -> Kd/1
  Kd/1 -> Sum/3  "D"
  Sum/1 -> Saturation/1
  Saturation/1 -> u/1

== system CCModel_73/Cruise Control/Version 3.0//3.1//3.2/Switches ==
  throttle_const : Inport
  t_out : Inport  Port=2
  brake_const : Inport  Port=3
  (False) : Constant  Value=0
  (True) : Constant
  Add Constant : Bias  Bias=5  SaturateOnIntegerOverflow=off
  Brake_Switch2 : Switch  Criteria=u2 > Threshold  SaturateOnIntegerOverflow=off  InputSameDT=off
  Constant : Constant  Value=0
  Constant3 : Constant  Value=0
  Gain : Gain
  Max : MinMax  Function=max  Inputs=2
  Max Throttle : Gain
  Pedal_threshold : Constant  Value=5
  Scope : Scope  NumInputPorts=2
  Subtract : Sum  Inputs=+-
  Switch : Switch  Criteria=u2 > Threshold  SaturateOnIntegerOverflow=off  InputSameDT=off
  Throttle_Switch : Switch  Criteria=u2 > Threshold  SaturateOnIntegerOverflow=off  InputSameDT=off
  Throttle_Switch2 : Switch  Criteria=u2 > Threshold  SaturateOnIntegerOverflow=off  InputSameDT=off
  Throttle : Outport
  Brake : Outport  Port=2
  Source : Outport  Port=3
  wires:
  throttle_const/1 -> Max/1, Throttle_Switch2/1
  brake_const/1 -> Max/2, Brake_Switch2/1
  Max/1 -> Subtract/1
  Pedal_threshold/1 -> Subtract/2
  Subtract/1 -> Switch/2
  (True)/1 -> Switch/1
  (False)/1 -> Switch/3
  Switch/1 -> Brake_Switch2/2, Throttle_Switch2/2, Source/1
  Constant3/1 -> Brake_Switch2/3
  Throttle_Switch/1 -> Add Constant/1
  Throttle_Switch2/1 -> Scope/2, Throttle/1
  Brake_Switch2/1 -> Brake/1
  Max Throttle/1 -> Throttle_Switch/1
  Constant/1 -> Throttle_Switch/3
  Add Constant/1 -> Gain/1
  t_out/1 -> Throttle_Switch/2, Max Throttle/1
  Gain/1 -> Throttle_Switch2/3

== system CCModel_73/Cruise Control/Version 3.0//3.1//3.2/Throttle ==
  New u : Inport
  Add3 : Sum
  Add4 : Sum
  Clock1 : Clock
  Delay : Delay  DelayLength=1
  Derivative : Derivative
  Gain : Gain  Gain=0.001
  Saturation1 : Saturate  UpperLimit=0  LowerLimit=0
  Saturation2 : Saturate  UpperLimit=0.025  LowerLimit=-0.025
  Saturation3 : Saturate  UpperLimit=60  LowerLimit=5
  Scope1 : Scope  NumInputPorts=2
  Scope2 : Scope  NumInputPorts=2
  Subtract1 : Sum  Inputs=-+
  Switch : Switch  Criteria=u2 > Threshold  SaturateOnIntegerOverflow=off  InputSameDT=off
  t_out : Outport
  wires:
  New u/1 -> Saturation3/1
  Derivative/1 -> Saturation1/1
  Saturation1/1 -> Gain/1
  Delay/1 -> Switch/1
  Gain/1 -> Add3/2
  Clock1/1 -> Switch/2
  Add3/1 -> Scope2/1, Add4/1, Subtract1/1
  Subtract1/1 -> Saturation2/1
  Saturation2/1 -> Scope2/2, Add4/2
  Add4/1 -> Scope1/2, Delay/1, t_out/1
  Saturation3/1 -> Subtract1/2, Switch/3, Scope1/1, Derivative/1
  Switch/1 -> Add3/1

== system CCModel_73/Cruise Control/Version 4.0/Detect Change ==
  note: This subsystem detects either a change in the reference velocity, or the driver releasing one of the pedals. It outputs the time of the change, the value of u just before the change, and a boolean "hasChanged" value
  desired_velocity : Inport
  throttle_const : Inport  Port=2
  brake_const : Inport  Port=3
  Smoothed u : Inport  Port=4
  (False) : Constant  Value=0
  (True) : Constant
  AND : Logic  IconShape=distinctive  AllPortsSameDT=off  OutDataTypeStr=boolean
  Clock : Clock
  Delay : Delay  DelayLength=1
  Detect Change : simulink/Logic and Bit Operations/Detect Change  vinit=0  OutDataTypeStr=boolean
  Detect Change1 : simulink/Logic and Bit Operations/Detect Change  vinit=0  OutDataTypeStr=boolean
  Max : MinMax  Function=max  Inputs=2
  OR : Logic  Operator=OR  IconShape=distinctive  AllPortsSameDT=off  OutDataTypeStr=boolean
  Pedal_threshold : Constant  Value=5
  Subtract : Sum  Inputs=+-
  Switch : Switch  Criteria=u2 > Threshold  SaturateOnIntegerOverflow=off  InputSameDT=off
  Switch1 : Switch  Criteria=u2 > Threshold  SaturateOnIntegerOverflow=off  InputSameDT=off
  Switch2 : Switch  Criteria=u2 > Threshold  SaturateOnIntegerOverflow=off  InputSameDT=off
  Change_time : Outport
  Old u : Outport  Port=2
  hasChanged : Outport  Port=3
  wires:
  desired_velocity/1 -> Detect Change/1
  Detect Change/1 -> OR/1
  OR/1 -> Switch/2, Switch2/2, hasChanged/1
  Switch1/1 -> Detect Change1/1, AND/1
  Detect Change1/1 -> AND/2
  AND/1 -> OR/2
  Clock/1 -> Switch/1
  Max/1 -> Subtract/1
  (True)/1 -> Switch1/1
  brake_const/1 -> Max/2
  Pedal_threshold/1 -> Subtract/2
  Subtract/1 -> Switch1/2
  (False)/1 -> Switch1/3
  throttle_const/1 -> Max/1
  Switch2/1 -> Switch2/3, Old u/1
  Delay/1 -> Switch2/1
  Switch/1 -> Switch/3, Change_time/1
  Smoothed u/1 -> Delay/1

== system CCModel_73/Cruise Control/Version 4.0/PID Controller ==
  note: Typical PID controller, outputs a value between -100 and 100
  error : Inport
  Derivative : Derivative
  Integrator : Integrator
  Kd : Gain  Gain=0.1
  Ki : Gain  Gain=0.03
  Kp : Gain  Gain=3
  Saturation : Saturate  UpperLimit=100  LowerLimit=-100
  Sum : Sum  Inputs=+++
  u : Outport
  wires:
  Integrator/1 -> Ki/1
  error/1 -> Integrator/1, Kp/1, Derivative/1  "D"
  Sum/1 -> Saturation/1
  Kp/1 -> Sum/2  "P"
  Ki/1 -> Sum/1  "I"
  Saturation/1 -> u/1
  Derivative/1 -> Kd/1
  Kd/1 -> Sum/3  "D"

== system CCModel_73/Cruise Control/Version 4.0/Sigmoid ==
  note: This whole part is just to eliminate weird cancellation errors that were happening
  note: This system smooths out curves using the sigmoid equation shown above.
      | u1 is "Old u" which is the last value u had when change was detected.
      | u2 is "New u" which is the current output being given by the PID controller.
      | x is the time elapsed since the last change
      | k is the "sigmoid gain" which dictates how fast the transition occurs
  Change_time : Inport
  Old u : Inport  Port=2
  New u : Inport  Port=3
  Add : Sum
  Add1 : Sum
  Add2 : Sum
  Clock : Clock
  Constant : Constant
  Constant1 : Constant
  Constant2 : Constant
  Divide : Product  Inputs=/*
  Divide1 : Product  Inputs=**
  Divide2 : Product  Inputs=/*
  Divide3 : Product  Inputs=**
  Gain : Gain  Gain=1000
  Gain1 : Gain  Gain=0.001
  K : Constant  Value=1.5
  Power{,1..3} (4 alike) : Math  Operator=pow
  Reciprocal : Product  Inputs=/
  Reciprocal1 : Product  Inputs=/
  Round : Rounding  Operator=round
  Scope : Scope  NumInputPorts=3
  Subtract : Sum  Inputs=-+
  Sum : Sum  Inputs=|-+
  u_out : Outport
  wires:
  Power1/1 -> Scope/3, Add/1
  Add/1 -> Power/1
  Clock/1 -> Sum/2
  Constant/1 -> Add/2
  Sum/1 -> Gain/1  "Elapsed Time"
  Reciprocal/1 -> Power/2
  Power/1 -> Divide/1
  Divide/1 -> Divide1/1  "Sigmoid Function"
  Add1/1 -> Power2/1
  Power3/1 -> Add1/1
  K/1 -> Scope/2, Reciprocal/1, Power1/2, Reciprocal1/1, Power3/2
  Reciprocal1/1 -> Power2/2
  Power2/1 -> Divide2/1
  Constant1/1 -> Add1/2
  Change_time/1 -> Sum/1
  Constant2/1 -> Subtract/2
  Divide2/1 -> Subtract/1  "Sigmoid Function"
  Divide1/1 -> Add2/1
  Add2/1 -> u_out/1
  New u/1 -> Divide1/2
  Old u/1 -> Divide3/2
  Subtract/1 -> Divide3/1
  Divide3/1 -> Add2/2
  Gain1/1 -> Power1/1, Divide/2, Scope/1, Divide2/2, Power3/1
  Gain/1 -> Round/1
  Round/1 -> Gain1/1

== system CCModel_73/Cruise Control/Version 4.0/Switches ==
  note: This subsystem determines the source of input, either the cruise control or the driver
      | It also determines for a given u if the brake or throttle should be applied
      | Lastly, it smooths out the cruise control brakes and throttles to prevent jerk peaks
  note: Apply sigmoid curving to the throttle and brake
  note: If u is positive, throttle is applied
      | If u is negative, brake is applied
      | Max gains prevent large jerks from happening
  note: If throttle or brake are above 5 the driver takes control of the system
  throttle_const : Inport
  u : Inport  Port=2
  brake_const : Inport  Port=3
  hasChanged : Inport  Port=4
  (False) : Constant  Value=0
  (True) : Constant
  Brake_Switch : Switch  Criteria=u2 > Threshold  SaturateOnIntegerOverflow=off  InputSameDT=off
  Brake_Switch2 : Switch  Criteria=u2 > Threshold  SaturateOnIntegerOverflow=off  InputSameDT=off
  Clock : Clock
  Clock1 : Clock
  Constant3 : Constant  Value=0
  Delay1 : Delay  DelayLength=1
  Delay3 : Delay  DelayLength=1
  Max : MinMax  Function=max  Inputs=2
  Max Brake : Gain  Gain=-0.5
  Max Throttle : Gain  Gain=0.8
  Pedal_threshold : Constant  Value=5
  Sigmoid_brake : Subsystem
  Sigmoid_throttle : Subsystem
  Subtract : Sum  Inputs=+-
  Switch : Switch  Criteria=u2 > Threshold  SaturateOnIntegerOverflow=off  InputSameDT=off
  Switch{1..4} (4 alike) : Switch  Criteria=u2 > Threshold  Threshold=0.04  SaturateOnIntegerOverflow=off  InputSameDT=off
  Throttle_Switch : Switch  Criteria=u2 > Threshold  SaturateOnIntegerOverflow=off  InputSameDT=off
  Throttle_Switch2 : Switch  Criteria=u2 > Threshold  SaturateOnIntegerOverflow=off  InputSameDT=off
  Throttle : Outport
  Brake : Outport  Port=2
  Source : Outport  Port=3
  wires:
  throttle_const/1 -> Throttle_Switch2/1, Max/1
  brake_const/1 -> Max/2, Brake_Switch2/1
  Max/1 -> Subtract/1
  Pedal_threshold/1 -> Subtract/2
  Subtract/1 -> Switch/2
  (True)/1 -> Switch/1
  (False)/1 -> Switch/3
  Switch/1 -> Brake_Switch2/2, Throttle_Switch2/2, Source/1
  u/1 -> Max Throttle/1, Throttle_Switch/2, Max Brake/1, Brake_Switch/2
  Constant3/1 -> Throttle_Switch/3, Brake_Switch/1
  Max Brake/1 -> Brake_Switch/3
  Throttle_Switch2/1 -> Throttle/1
  Brake_Switch2/1 -> Brake/1
  Max Throttle/1 -> Throttle_Switch/1
  Switch1/1 -> Switch1/3, Sigmoid_throttle/1(Change_time)  "Time"
  Switch2/1 -> Switch2/3, Sigmoid_throttle/2(Old thr)  "Old throttle"
  Throttle_Switch/1 -> Sigmoid_throttle/3(New thr)  "Throttle"
  Sigmoid_throttle/1(throttle_out) -> Delay1/1, Throttle_Switch2/3  "Smoothed throttle"
  Clock/1 -> Switch1/1
  hasChanged/1 -> Switch4/2, Switch3/2, Switch1/2, Switch2/2
  Delay1/1 -> Switch2/1
  Switch3/1 -> Switch3/3, Sigmoid_brake/1(Change_time)  "Time"
  Brake_Switch/1 -> Sigmoid_brake/3(New brake)  "Brake"
  Clock1/1 -> Switch3/1
  Switch4/1 -> Switch4/3, Sigmoid_brake/2(Old brake)  "Old brake"
  Delay3/1 -> Switch4/1
  Sigmoid_brake/1(brake_out) -> Delay3/1, Brake_Switch2/3  "Smoothed Brake"
